simulink model "Rectifier_sim_model"  (R2016a)
settings: Solver=ode4  StartTime=0.0  StopTime=Tfinal  FixedStep=Ts  RelTol=1e-3
values from neighbouring files (symbols this model uses):
  Cdc = 15e-6    (= 1.5e-05)    [balancing_sim_parameters.m]    (also in rectifier_sim_parameters.m; sixthharmonicstudies_another_sim_param.m)
  Cdcrec = 4e-3    (= 0.004)    [balancing_sim_parameters.m]    (also in rectifier_sim_parameters.m = 0.0011; sixthharmonicstudies_another_sim_param.m)
  delta = 0    [balancing_sim_parameters.m]    (also in rectifier_sim_parameters.m; sixthharmonicstudies_another_sim_param.m = 2.09439510239)
  delta_third = 0*pi/180    (= 0)    [rectifier_sim_parameters.m]
  ESLrec = 100e-9    (= 1e-07)    [rectifier_sim_parameters.m]
  ESRrec = 10e-3    (= 0.01)    [rectifier_sim_parameters.m]
  f_third = 150    [rectifier_sim_parameters.m]
  GridFreq = 50    [balancing_sim_parameters.m]    (also in rectifier_sim_parameters.m; sixthharmonicstudies_another_sim_param.m)
  Is1_f = 150    [rectifier_sim_parameters.m]
  Is3_f = 150    [rectifier_sim_parameters.m]
  Isa1 = 10    [rectifier_sim_parameters.m]
  Isa1_delta = 0*pi/180    (= 0)    [rectifier_sim_parameters.m]
  Isa3 = third    (= 0)    [rectifier_sim_parameters.m]
  Isa3_delta = 0*pi/180    (= 0)    [rectifier_sim_parameters.m]
  Isb1 = 5    [rectifier_sim_parameters.m]
  Isb1_delta = -120*pi/180    (= -2.09439510239)    [rectifier_sim_parameters.m]
  Isb3 = third    (= 0)    [rectifier_sim_parameters.m]
  Isb3_delta = 0*pi/180    (= 0)    [rectifier_sim_parameters.m]
  Isc1 = 5    [rectifier_sim_parameters.m]
  Isc1_delta = 120*pi/180    (= 2.09439510239)    [rectifier_sim_parameters.m]
  Isc3 = third    (= 0)    [rectifier_sim_parameters.m]
  Isc3_delta = 0*pi/180    (= 0)    [rectifier_sim_parameters.m]
  Lload_1A = Lnom*1.00    [balancing_sim_parameters.m]    (also in rectifier_sim_parameters.m; sixthharmonicstudies_another_sim_param.m)
  Lload_1B = Lnom*1.00    [balancing_sim_parameters.m]    (also in rectifier_sim_parameters.m; sixthharmonicstudies_another_sim_param.m)
  Lload_1C = Lnom*1.00    [balancing_sim_parameters.m]    (also in rectifier_sim_parameters.m; sixthharmonicstudies_another_sim_param.m)
  Lmid = 1e-6    (= 1e-06)    [rectifier_sim_parameters.m]
  ma1 = 0.9    [balancing_sim_parameters.m]    (also in balancing_voltage_calc.m; rectifier_sim_parameters.m; sixthharmonicstudies_another_sim_param.m)
  ma_third = 0.5    [rectifier_sim_parameters.m]
  phase = [0 90 0 90]    [balancing_sim_parameters.m]    (also in rectifier_sim_parameters.m; sixthharmonicstudies_another_sim_param.m)
  Rin = 0    [balancing_sim_parameters.m]    (also in rectifier_sim_parameters.m = 10; sixthharmonicstudies_another_sim_param.m = 10)
  Ripth = 0.18    [balancing_sim_parameters.m]    (also in rectifier_sim_parameters.m; sixthharmonicstudies_another_sim_param.m)
  Rload_1A = Rnom*1.00    [balancing_sim_parameters.m]    (also in rectifier_sim_parameters.m; sixthharmonicstudies_another_sim_param.m)
  Rload_1B = Rnom*1.00    [balancing_sim_parameters.m]    (also in rectifier_sim_parameters.m; sixthharmonicstudies_another_sim_param.m = Rnom*2.5)
  Rload_1C = Rnom*1.00    [balancing_sim_parameters.m]    (also in rectifier_sim_parameters.m; sixthharmonicstudies_another_sim_param.m = Rnom*2.5)
  Rmid = 4    [balancing_sim_parameters.m]    (also in rectifier_sim_parameters.m = 3; sixthharmonicstudies_another_sim_param.m = 0.1)
  SA_delta1 = 0*pi/180    (= 0)    [rectifier_sim_parameters.m]
  SA_delta3 = 0*pi/180    (= 0)    [rectifier_sim_parameters.m]
  SA_f1 = 150    [rectifier_sim_parameters.m]
  SA_f3 = 150    [rectifier_sim_parameters.m]
  SA_ma1 = 0.9    [rectifier_sim_parameters.m]
  SA_ma3 = 0    [rectifier_sim_parameters.m]
  SB_delta3 = 0*pi/180    (= 0)    [rectifier_sim_parameters.m]
  SC_delta3 = 0*pi/180    (= 0)    [rectifier_sim_parameters.m]
  Ts = 1e-7    (= 1e-07)    [balancing_sim_parameters.m]    (also in rectifier_sim_parameters.m = 1e-06; sixthharmonicstudies_another_sim_param.m = 1e-06)
  Vacrms = 140    [balancing_sim_parameters.m]    (also in rectifier_sim_parameters.m = 120; sixthharmonicstudies_another_sim_param.m = 115)
  Vin = Vdc + Rin*(Pout/Vdc)+3    (= 1310.03703704)    [balancing_sim_parameters.m]    (also in rectifier_sim_parameters.m = 366.296296296; sixthharmonicstudies_another_sim_param.m = 344.814814815)
  wout = 2*pi*fout    (= 314.159265359)    [balancing_sim_parameters.m]    (also in rectifier_sim_parameters.m; sixthharmonicstudies_another_sim_param.m = 942.477796077)
undefined symbols (not defined in the file or in its folder): GridPhase, Lload, Rload, SA_delta, SA_f, SA_ma
libraries: powerlib x89, powerlib_meascontrol x63, simulink x6
settings Model: SimulationMode=accelerator  Creator=ugurm  LastModifiedBy=mesutto
settings DataIOCC: LimitDataPoints=on  SaveFormat=Array
settings DebuggingCC: UnderspecifiedInitializationDetection=Classic  MergeDetectMultiDrivingBlocksExec=none  SolverPrmCheckMsg=warning  StateNameClashWarn=warning
settings HardwareCC: ProdBitPerPointer=32  ProdLargestAtomicFloat=None  ProdIntDivRoundTo=Undefined  ProdEndianess=Unspecified  ProdWordSize=32  ProdHWDeviceType=32-bit Generic
settings ModelReferenceCC: PropagateSignalLabelsOutOfModel=off
settings ConfigComp: CovModelRefEnable=Off

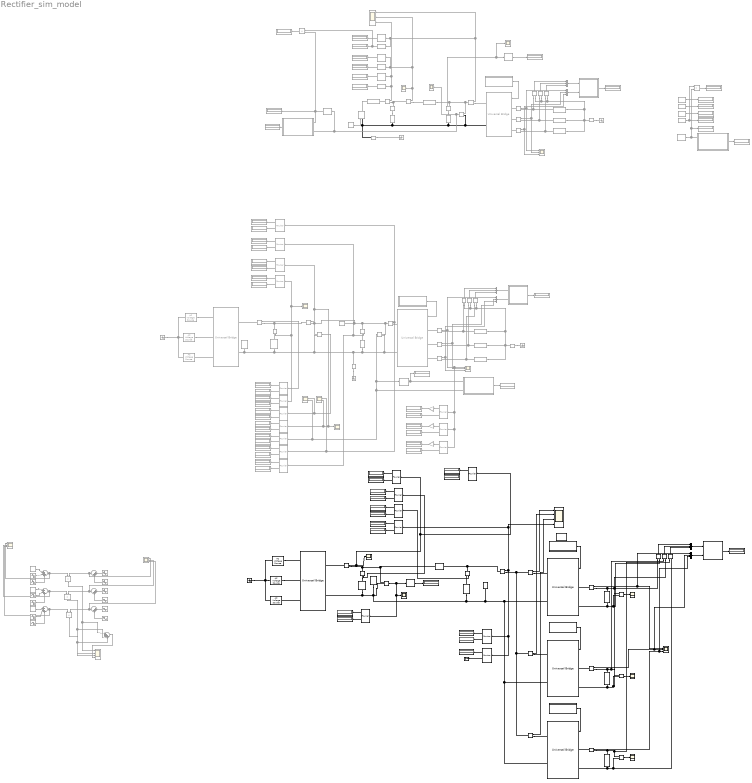
== system Rectifier_sim_model ==
  note: Iinput
  note: Idc
  note: Icap
  note: Vdc
  note: Vinput
  note: Ireccap
  note: Irec
  AC Voltage Source1 : powerlib/Electrical Sources/AC Voltage Source  Commented=on  Amplitude=Vacrms*sqrt(2)  Phase=-120  Frequency=GridFreq  SampleTime=0  Measurements=None  BusType=swing  Pref=10e3  Qref=0  Qmin=-inf  Qmax=+inf
  AC Voltage Source2 : powerlib/Electrical Sources/AC Voltage Source  Commented=on  Amplitude=Vacrms*sqrt(2)  Phase=0  Frequency=GridFreq  SampleTime=0  Measurements=None  BusType=swing  Pref=10e3  Qref=0  Qmin=-inf  Qmax=+inf
  AC Voltage Source3 : powerlib/Electrical Sources/AC Voltage Source  Commented=on  Amplitude=Vacrms*sqrt(2)  Phase=-240  Frequency=GridFreq  SampleTime=0  Measurements=None  BusType=swing  Pref=10e3  Qref=0  Qmin=-inf  Qmax=+inf
  AC Voltage Source4 : powerlib/Electrical Sources/AC Voltage Source  Amplitude=Vacrms*sqrt(2)  Phase=-120+GridPhase  Frequency=GridFreq  SampleTime=0  Measurements=None  BusType=swing  Pref=10e3  Qref=0  Qmin=-inf  Qmax=+inf
  AC Voltage Source5 : powerlib/Electrical Sources/AC Voltage Source  Amplitude=Vacrms*sqrt(2)  Phase=GridPhase  Frequency=GridFreq  SampleTime=0  Measurements=None  BusType=swing  Pref=10e3  Qref=0  Qmin=-inf  Qmax=+inf
  AC Voltage Source6 : powerlib/Electrical Sources/AC Voltage Source  Amplitude=Vacrms*sqrt(2)  Phase=-240+GridPhase  Frequency=GridFreq  SampleTime=0  Measurements=None  BusType=swing  Pref=10e3  Qref=0  Qmin=-inf  Qmax=+inf
  Constant : Constant  Commented=on  Value=1/2
  Constant1 : Constant  Commented=on  Value=Vin
  Constant2 : Constant  Commented=on  Value=1/2
  Constant3 : Constant  Commented=on  Value=1/2
  DC Voltage Source : powerlib/Electrical Sources/DC Voltage Source  Amplitude=270  Measurements=None
  Display{,1..48} (49 alike) : Display  Commented=on
  Display{49..65} (17 alike) : Display
  Fourier1 : powerlib_meascontrol/Measurements/Fourier  Commented=on  Freq=50  n=5  InInit=[0, 0]  Ts=0
  Fourier{8..11} (4 alike) : powerlib_meascontrol/Measurements/Fourier  Commented=on  Freq=9850  n=1  InInit=[0, 0]  Ts=0
  Fourier12 : powerlib_meascontrol/Measurements/Fourier  Commented=on  Freq=50  n=3  InInit=[0, 0]  Ts=0
  Fourier{2..6,13..14} (7 alike) : powerlib_meascontrol/Measurements/Fourier  Commented=on  Freq=50  n=6  InInit=[0, 0]  Ts=0
  Fourier{15,17..20,22} (6 alike) : powerlib_meascontrol/Measurements/Fourier  Freq=50  n=6  InInit=[0, 0]  Ts=0
  Fourier16 : powerlib_meascontrol/Measurements/Fourier  Freq=50  n=0  InInit=[0, 0]  Ts=0
  Fourier21 : powerlib_meascontrol/Measurements/Fourier  Freq=50  n=0  InInit=[0, 0]  Ts=0
  Fourier7 : powerlib_meascontrol/Measurements/Fourier  Commented=on  Freq=50  n=7  InInit=[0, 0]  Ts=0
  Gain : Gain  Commented=on  Gain=100
  Gain1 : Gain  Commented=on  Gain=100
  Gain2 : Gain  Commented=on  Gain=100
  Gate drive 1 : Subsystem  Commented=on
  Gate drive 2 : Subsystem
  Gate drive 3 : Subsystem
  Gate drive 4 : Subsystem
  Gate drive 5 : Subsystem  Commented=on
  Ground{1..3,5..6} (5 alike) : powerlib/Elements/Ground  Commented=on  LConnTagsString=a
  Ground4 : powerlib/Elements/Ground  LConnTagsString=a
  Idc_m{1..11,14..17,19} (16 alike) : powerlib/Measurements/Current Measurement  Commented=on  PhasorSimulation=off  OutputType=Complex  PSBequivalent=0
  Idc_m{12..13,18,20..26} (10 alike) : powerlib/Measurements/Current Measurement  PhasorSimulation=off  OutputType=Complex  PSBequivalent=0
  Mean{,1..7} (8 alike) : powerlib_meascontrol/Measurements/Mean  Commented=on  Freq=fout  Vinit=0  Ts=0
  Mean8 : powerlib_meascontrol/Measurements/Mean  Freq=50  Vinit=0  Ts=0
  Mux{,1..3} (4 alike) : Mux  Commented=on  Inputs=3
  Mux4 : Mux  Inputs=3
  Mux5 : Mux  Inputs=3
  Product{,1..4} (5 alike) : Product  Commented=on
  RMS{1..6} (6 alike) : powerlib_meascontrol/Measurements/RMS  Commented=on  TrueRMS=on  Freq=fout  RMSInit=0  Ts=0
  Scope{,2..5} (5 alike) : Scope  Commented=on
  Scope{1,6,8..10} (5 alike) : Scope  Commented=on  NumInputPorts=3
  Scope11 : Scope  Commented=on  NumInputPorts=2
  Scope12 : Scope  Commented=on  NumInputPorts=4
  Scope{13,16..19} (5 alike) : Scope
  Scope14 : Scope  NumInputPorts=3
  Scope15 : Scope  NumInputPorts=4
  Scope7 : Scope  Commented=on  NumInputPorts=2
  Series RLC Branch1 : powerlib/Elements/Series RLC Branch  Commented=on  LConnTagsString=__new0  RConnTagsString=__new0  BranchType=RL  Resistance=Rload_1B  Inductance=Lload_1B  SetiL0=off  InitialCurrent=0  Capacitance=1e-6  Setx0=off  InitialVoltage=0  Measurements=None
  Series RLC Branch{10,14,40,42} (4 alike) : powerlib/Elements/Series RLC Branch  Commented=on  LConnTagsString=__new0  RConnTagsString=__new0  BranchType=R  Resistance=1e12  Inductance=Lload  SetiL0=off  InitialCurrent=0  Capacitance=1e-6  Setx0=off  InitialVoltage=0  Measurements=None
  Series RLC Branch11 : powerlib/Elements/Series RLC Branch  Commented=on  LConnTagsString=__new0  RConnTagsString=__new0  BranchType=RL  Resistance=Rload_1A  Inductance=Lload_1A  SetiL0=off  InitialCurrent=0  Capacitance=1e-6  Setx0=off  InitialVoltage=0  Measurements=None
  Series RLC Branch12 : powerlib/Elements/Series RLC Branch  Commented=on  LConnTagsString=__new0  RConnTagsString=__new0  BranchType=C  Resistance=Rload  Inductance=Lload  SetiL0=off  InitialCurrent=0  Capacitance=Cdc  Setx0=off  InitialVoltage=0  Measurements=None
  Series RLC Branch13 : powerlib/Elements/Series RLC Branch  Commented=on  LConnTagsString=__new0  RConnTagsString=__new0  BranchType=RL  Resistance=Rmid  Inductance=Lmid  SetiL0=off  InitialCurrent=0  Capacitance=1e-6  Setx0=off  InitialVoltage=0  Measurements=None
  Series RLC Branch15 : powerlib/Elements/Series RLC Branch  LConnTagsString=__new0  RConnTagsString=__new0  BranchType=RL  Resistance=Rload_1A  Inductance=Lload_1A  SetiL0=off  InitialCurrent=0  Capacitance=1e-6  Setx0=off  InitialVoltage=0  Measurements=None
  Series RLC Branch16 : powerlib/Elements/Series RLC Branch  LConnTagsString=__new0  RConnTagsString=__new0  BranchType=R  Resistance=Rmid  Inductance=1e-6  SetiL0=off  InitialCurrent=0  Capacitance=Cdcrec  Setx0=on  InitialVoltage=270  Measurements=None
  Series RLC Branch17 : powerlib/Elements/Series RLC Branch  LConnTagsString=__new0  RConnTagsString=__new0  BranchType=C  Resistance=ESRrec  Inductance=ESLrec  SetiL0=off  InitialCurrent=0  Capacitance=Cdc  Setx0=off  InitialVoltage=270  Measurements=None
  Series RLC Branch18 : powerlib/Elements/Series RLC Branch  LConnTagsString=__new0  RConnTagsString=__new0  BranchType=R  Resistance=36.5  Inductance=ESLrec  SetiL0=off  InitialCurrent=0  Capacitance=Cdcrec  Setx0=on  InitialVoltage=270  Measurements=None
  Series RLC Branch19 : powerlib/Elements/Series RLC Branch  LConnTagsString=__new0  RConnTagsString=__new0  BranchType=C  Resistance=ESRrec  Inductance=ESLrec  SetiL0=off  InitialCurrent=0  Capacitance=Cdcrec  Setx0=on  InitialVoltage=270  Measurements=None
  Series RLC Branch2 : powerlib/Elements/Series RLC Branch  Commented=on  LConnTagsString=__new0  RConnTagsString=__new0  BranchType=RL  Resistance=Rload_1C  Inductance=Lload_1C  SetiL0=off  InitialCurrent=0  Capacitance=1e-6  Setx0=off  InitialVoltage=0  Measurements=None
  Series RLC Branch20 : powerlib/Elements/Series RLC Branch  Commented=on  LConnTagsString=__new0  RConnTagsString=__new0  BranchType=R  Resistance=Rin  Inductance=1e-3  SetiL0=off  InitialCurrent=0  Capacitance=1e-6  Setx0=off  InitialVoltage=0  Measurements=None
  Series RLC Branch21 : powerlib/Elements/Series RLC Branch  Commented=on  LConnTagsString=__new0  RConnTagsString=__new0  BranchType=C  Resistance=Rload  Inductance=Lload  SetiL0=off  InitialCurrent=0  Capacitance=Cdc  Setx0=off  InitialVoltage=0  Measurements=None
  Series RLC Branch22 : powerlib/Elements/Series RLC Branch  LConnTagsString=__new0  RConnTagsString=__new0  BranchType=RL  Resistance=Rload_1A  Inductance=Lload_1A  SetiL0=off  InitialCurrent=0  Capacitance=1e-6  Setx0=off  InitialVoltage=0  Measurements=None
  Series RLC Branch23 : powerlib/Elements/Series RLC Branch  LConnTagsString=__new0  RConnTagsString=__new0  BranchType=RL  Resistance=Rload_1A  Inductance=Lload_1A  SetiL0=off  InitialCurrent=0  Capacitance=1e-6  Setx0=off  InitialVoltage=0  Measurements=None
  Series RLC Branch3 : powerlib/Elements/Series RLC Branch  Commented=on  LConnTagsString=__new0  RConnTagsString=__new0  BranchType=C  Resistance=Rload  Inductance=Lload  SetiL0=off  InitialCurrent=0  Capacitance=Cdcrec  Setx0=on  InitialVoltage=270  Measurements=None
  Series RLC Branch4 : powerlib/Elements/Series RLC Branch  Commented=on  LConnTagsString=__new0  RConnTagsString=__new0  BranchType=R  Resistance=Rmid  Inductance=1e-3  SetiL0=off  InitialCurrent=0  Capacitance=1e-6  Setx0=off  InitialVoltage=0  Measurements=None
  Series RLC Branch5 : powerlib/Elements/Series RLC Branch  Commented=on  LConnTagsString=__new0  RConnTagsString=__new0  BranchType=RLC  Resistance=ESRrec  Inductance=ESLrec  SetiL0=off  InitialCurrent=0  Capacitance=Cdcrec  Setx0=on  InitialVoltage=270  Measurements=None
  Series RLC Branch6 : powerlib/Elements/Series RLC Branch  Commented=on  LConnTagsString=__new0  RConnTagsString=__new0  BranchType=RL  Resistance=Rload_1A  Inductance=Lload_1A  SetiL0=off  InitialCurrent=0  Capacitance=1e-6  Setx0=off  InitialVoltage=0  Measurements=None
  Series RLC Branch7 : powerlib/Elements/Series RLC Branch  Commented=on  LConnTagsString=__new0  RConnTagsString=__new0  BranchType=C  Resistance=ESRrec  Inductance=ESLrec  SetiL0=off  InitialCurrent=0  Capacitance=Cdcrec  Setx0=on  InitialVoltage=270  Measurements=None
  Series RLC Branch8 : powerlib/Elements/Series RLC Branch  Commented=on  LConnTagsString=__new0  RConnTagsString=__new0  BranchType=RL  Resistance=Rload_1B  Inductance=Lload_1B  SetiL0=off  InitialCurrent=0  Capacitance=1e-6  Setx0=off  InitialVoltage=0  Measurements=None
  Series RLC Branch9 : powerlib/Elements/Series RLC Branch  Commented=on  LConnTagsString=__new0  RConnTagsString=__new0  BranchType=RL  Resistance=Rload_1C  Inductance=Lload_1C  SetiL0=off  InitialCurrent=0  Capacitance=1e-6  Setx0=off  InitialVoltage=0  Measurements=None
  Sine Wave : Sin  Commented=on  Amplitude=Isa1  Frequency=Is1_f*2*pi  Phase=Isa1_delta  SampleTime=0
  Sine Wave1 : Sin  Commented=on  Amplitude=SA_ma1/2  Frequency=SA_f1*2*pi  Phase=SA_delta1  SampleTime=0
  Sine Wave10 : Sin  Commented=on  Amplitude=SA_ma3/2  Frequency=SA_f3*2*pi  Phase=SB_delta3  SampleTime=0
  Sine Wave11 : Sin  Commented=on  Amplitude=SA_ma3/2  Frequency=SA_f3*2*pi  Phase=SC_delta3  SampleTime=0
  Sine Wave2 : Sin  Commented=on  Amplitude=SA_ma1/2  Frequency=SA_f1*2*pi  Phase=SA_delta1-2*pi/3  SampleTime=0
  Sine Wave3 : Sin  Commented=on  Amplitude=Isa3  Frequency=Is3_f*2*pi  Phase=Isa3_delta  SampleTime=0
  Sine Wave4 : Sin  Commented=on  Amplitude=SA_ma/2  Frequency=SA_f*2*pi  Phase=SA_delta+2*pi/3  SampleTime=0
  Sine Wave5 : Sin  Commented=on  Amplitude=Isb1  Frequency=Is1_f*2*pi  Phase=Isb1_delta  SampleTime=0
  Sine Wave6 : Sin  Commented=on  Amplitude=Isb3  Frequency=Is3_f*2*pi  Phase=Isb3_delta  SampleTime=0
  Sine Wave7 : Sin  Commented=on  Amplitude=Isc1  Frequency=Is1_f*2*pi  Phase=Isc1_delta  SampleTime=0
  Sine Wave8 : Sin  Commented=on  Amplitude=Isc3  Frequency=Is3_f*2*pi  Phase=Isc3_delta  SampleTime=0
  Sine Wave9 : Sin  Commented=on  Amplitude=SA_ma3/2  Frequency=SA_f3*2*pi  Phase=SA_delta3  SampleTime=0
  Subsystem1 : Subsystem  Commented=on
  Subsystem2 : Subsystem  Commented=on
  Subsystem3 : Subsystem  Commented=on
  Subsystem4 : Subsystem  Commented=on
  Subsystem5 : Subsystem  Commented=on
  Subsystem6 : Subsystem
  Sum{1..2,4,7} (4 alike) : Sum  Commented=on  Inputs=|+++
  Sum3 : Sum  Commented=on  Inputs=|++
  Sum5 : Sum  Commented=on  Inputs=|++
  Sum6 : Sum  Commented=on  Inputs=|++
  Terminator : Terminator
  Universal Bridge1 : powerlib/Power Electronics/Universal Bridge  Commented=on  Arms=3  SnubberResistance=1e5  SnubberCapacitance=inf  Device=Diodes  Ron=1e-6  Lon=0  ForwardVoltages="[  0  0  ]"  ForwardVoltage=0  GTOparameters=[ 10e-6 , 20e-6 ]  IGBTparameters=[0,0]  Measurements=None  Measurements_2=None  converterType=Rectifier
  Universal Bridge2 : powerlib/Power Electronics/Universal Bridge  Commented=on  Arms=3  SnubberResistance=1e5  SnubberCapacitance=inf  Device=IGBT / Diodes  Ron=1e-6  Lon=0  ForwardVoltages="[  0  0  ]"  ForwardVoltage=0  GTOparameters=[ 10e-6 , 20e-6 ]  IGBTparameters=[0,0]  Measurements=None  Measurements_2=None  converterType=Rectifier
  Universal Bridge3 : powerlib/Power Electronics/Universal Bridge  Arms=2  SnubberResistance=1e5  SnubberCapacitance=inf  Device=IGBT / Diodes  Ron=1e-6  Lon=0  ForwardVoltages="[  0  0  ]"  ForwardVoltage=0  GTOparameters=[ 10e-6 , 20e-6 ]  IGBTparameters=[0,0]  Measurements=None  Measurements_2=None  converterType=Rectifier
  Universal Bridge4 : powerlib/Power Electronics/Universal Bridge  Commented=on  Arms=3  SnubberResistance=1e5  SnubberCapacitance=inf  Device=IGBT / Diodes  Ron=1e-6  Lon=0  ForwardVoltages="[  0  0  ]"  ForwardVoltage=0  GTOparameters=[ 10e-6 , 20e-6 ]  IGBTparameters=[0,0]  Measurements=None  Measurements_2=None  converterType=Rectifier
  Universal Bridge5 : powerlib/Power Electronics/Universal Bridge  Arms=2  SnubberResistance=1e5  SnubberCapacitance=inf  Device=IGBT / Diodes  Ron=1e-6  Lon=0  ForwardVoltages="[  0  0  ]"  ForwardVoltage=0  GTOparameters=[ 10e-6 , 20e-6 ]  IGBTparameters=[0,0]  Measurements=None  Measurements_2=None  converterType=Rectifier
  Universal Bridge6 : powerlib/Power Electronics/Universal Bridge  Arms=2  SnubberResistance=1e5  SnubberCapacitance=inf  Device=IGBT / Diodes  Ron=1e-6  Lon=0  ForwardVoltages="[  0  0  ]"  ForwardVoltage=0  GTOparameters=[ 10e-6 , 20e-6 ]  IGBTparameters=[0,0]  Measurements=None  Measurements_2=None  converterType=Rectifier
  Universal Bridge7 : powerlib/Power Electronics/Universal Bridge  Arms=3  SnubberResistance=1e5  SnubberCapacitance=inf  Device=Diodes  Ron=1e-6  Lon=0  ForwardVoltages="[  0  0  ]"  ForwardVoltage=0  GTOparameters=[ 10e-6 , 20e-6 ]  IGBTparameters=[0,0]  Measurements=None  Measurements_2=None  converterType=Rectifier
  Vdc1 : powerlib/Electrical Sources/Controlled Voltage Source  Commented=on  Initialize=off  Source_Type=DC  Amplitude=200  Phase=0  Frequency=0  Measurements=None
  Vdc_m{1..9} (9 alike) : powerlib/Measurements/Voltage Measurement  Commented=on  PhasorSimulation=off  OutputType=Complex  PSBequivalent=0
  Vdc_m{10..15} (6 alike) : powerlib/Measurements/Voltage Measurement  PhasorSimulation=off  OutputType=Complex  PSBequivalent=0
  Voltage Measurement : powerlib/Measurements/Voltage Measurement  PhasorSimulation=off  OutputType=Complex  PSBequivalent=0
  powergui1 : powerlib/powergui  Priority=1  SimulationMode=Discrete  SolverType=Tustin  SampleTime=Ts  frequency=60  SPID=off  DisableSnubberDevices=off  DisableRonSwitches=off  DisableVfSwitches=off  SwTol=0  DisplayEquations=off  Interpol=off  ExternalGateDelay=off  methode=off  Ts=0  FunctionMessages=off  echomessages=off  HookPort=off  EnableUseOfTLC=off  x0status=blocks  frequencyindice=0  Pbase=100e6  ErrMax=1e-4  Iterations=50  UnitsV=kV  UnitsW=MW  buscounter=0  RestoreLinks=warning  ResistiveCurrentMeasurement=off  Frange=[0:2:500]  Ylog=off  Xlog=on  ShowGrid=off  save=off  variable=ZData  structure=newidcs  ZoomFFT=off  StartTime=0.04  cycles=5  DisplayStyle=5  fundamental=50  FreqAxis=off  MaxFrequency=2000  frequencyindicesteady=1  RmsSteady=1  display=off
  wires:
  Gate drive 5/1(gate1) -> Universal Bridge4/1
  Idc_m14/1 -> Mux1/1, Scope8/1
  Constant1/1 -> Vdc1/1
  Idc_m15/1 -> RMS3/1, Scope3/1
  Idc_m16/1 -> Mux1/2, Scope8/2
  Idc_m17/1 -> Scope8/3, Mux1/3
  RMS3/1 -> Display/1
  Mean/1 -> Product/2, Subsystem5/1(Vdcavg), Display8/1
  RMS2/1 -> Display4/1
  Idc_m11/1 -> Scope1/1, RMS2/1, Mean3/1
  Idc_m19/1 -> Scope2/1, Scope1/2, Mean6/1, RMS5/1
  Mean3/1 -> Product/1, Display7/1
  RMS5/1 -> Display12/1
  Mean6/1 -> Display11/1
  Subsystem5/1(Out1) -> Display14/1
  Product/1 -> Display17/1
  Vdc_m5/1 -> Mux/1
  Vdc_m2/1 -> Mux/2
  Vdc_m6/1 -> Mux/3
  Mux/1 -> Subsystem4/1(Vabc)
  Mux1/1 -> Subsystem4/2(Iabc)
  Subsystem4/1(Poutp) -> Display20/1
  Vdc_m1/1 -> Scope4/1, Mean/1, Subsystem5/2(vdc)
  Idc_m2/1 -> Mean1/1, Scope1/3, RMS1/1
  Mean1/1 -> Display1/1
  RMS1/1 -> Display2/1
  Idc_m4/1 -> Fourier9/1, Scope11/2, Fourier3/1, Scope/1
  Vdc_m3/1 -> Fourier2/1, Scope7/1
  Mean5/1 -> Display15/1, Product1/2, Subsystem1/1(Vdcavg)
  Subsystem1/1(Out1) -> Display3/1
  RMS4/1 -> Display5/1
  Mean2/1 -> Display6/1
  Mean4/1 -> Product1/1, Display10/1
  RMS6/1 -> Display9/1
  Product1/1 -> Display13/1
  Gate drive 1/1(gate1) -> Universal Bridge2/1
  Idc_m6/1 -> Mux3/1, Fourier12/1, Fourier7/1, Fourier1/1, Scope9/1
  Idc_m7/1 -> Mux3/2, Scope9/2
  Idc_m8/1 -> Mux3/3, Scope9/3
  Vdc_m8/1 -> Mux2/1
  Vdc_m7/1 -> Mux2/2
  Vdc_m9/1 -> Mux2/3
  Mux2/1 -> Subsystem2/1(Vabc)
  Mux3/1 -> Subsystem2/2(Iabc)
  Subsystem2/1(Poutp) -> Display18/1
  Vdc_m4/1 -> Fourier4/1, Scope7/2, Subsystem3/2(vdc), Mean7/1
  Mean7/1 -> Subsystem3/1(Vdcavg), Display16/1
  Subsystem3/1(Out1) -> Display19/1
  Fourier2/1 -> Display25/1
  Fourier2/2 -> Display26/1
  Fourier3/1 -> Display27/1
  Fourier3/2 -> Display28/1
  Fourier4/1 -> Display29/1
  Fourier4/2 -> Display30/1
  Fourier5/1 -> Display31/1
  Fourier5/2 -> Display32/1
  Fourier6/1 -> Display33/1
  Fourier6/2 -> Display34/1
  Fourier1/1 -> Gain/1
  Fourier1/2 -> Display22/1
  Fourier7/1 -> Gain1/1
  Fourier7/2 -> Display24/1
  Fourier8/1 -> Display35/1
  Fourier8/2 -> Display36/1
  Fourier9/1 -> Display37/1
  Fourier9/2 -> Display38/1
  Idc_m10/1 -> Fourier10/1, Fourier6/1
  Fourier10/1 -> Display39/1
  Fourier10/2 -> Display40/1
  Idc_m5/1 -> Fourier5/1, Scope11/1, Fourier11/1
  Fourier11/1 -> Display41/1
  Fourier11/2 -> Display42/1
  Fourier12/1 -> Gain2/1
  Fourier12/2 -> Display44/1
  Gain/1 -> Display21/1
  Gain1/1 -> Display23/1
  Gain2/1 -> Display43/1
  Idc_m3/1 -> Scope5/1, Fourier8/1, Fourier14/1
  Idc_m9/1 -> Fourier13/1
  Fourier13/1 -> Display45/1
  Fourier13/2 -> Display46/1
  Fourier14/1 -> Display47/1
  Fourier14/2 -> Display48/1
  Sine Wave/1 -> Sum3/1
  Sine Wave3/1 -> Sum3/2
  Constant/1 -> Sum1/1
  Sine Wave1/1 -> Sum1/2
  Constant2/1 -> Sum2/1
  Sine Wave2/1 -> Sum2/2
  Constant3/1 -> Sum4/1
  Sine Wave4/1 -> Sum4/2
  Sine Wave5/1 -> Sum5/1
  Sine Wave6/1 -> Sum5/2
  Sine Wave7/1 -> Sum6/1
  Sine Wave8/1 -> Sum6/2
  Sum2/1 -> Product3/1, Scope6/2
  Sum1/1 -> Product2/1, Scope6/1
  Sum5/1 -> Product3/2, Scope10/2
  Sum3/1 -> Product2/2, Scope10/1
  Sum4/1 -> Product4/1, Scope6/3
  Sum6/1 -> Product4/2, Scope10/3
  Product2/1 -> Sum7/1, Scope12/1
  Product3/1 -> Scope12/2, Sum7/2
  Product4/1 -> Scope12/3, Sum7/3
  Sum7/1 -> Scope12/4
  Sine Wave9/1 -> Sum1/3
  Sine Wave10/1 -> Sum2/3
  Sine Wave11/1 -> Sum4/3
  Gate drive 2/1(gate1) -> Universal Bridge3/1
  Vdc_m10/1 -> Scope13/1
  Gate drive 3/1(gate1) -> Universal Bridge5/1
  Vdc_m11/1 -> Scope16/1
  Gate drive 4/1(gate1) -> Universal Bridge6/1
  Vdc_m12/1 -> Scope18/1
  Idc_m13/1 -> Scope15/1
  Idc_m21/1 -> Scope15/2
  Idc_m22/1 -> Scope15/3
  Idc_m23/1 -> Scope15/4, Fourier19/1, Fourier16/1, Fourier15/1
  Fourier15/1 -> Display49/1
  Fourier15/2 -> Display50/1
  Fourier16/1 -> Display51/1
  Fourier16/2 -> Terminator/1
  Fourier17/1 -> Display52/1
  Fourier17/2 -> Display53/1
  Fourier18/1 -> Display54/1
  Fourier18/2 -> Display55/1
  Voltage Measurement/1 -> Mean8/1, Scope19/1, Fourier18/1
  Mean8/1 -> Display56/1
  Fourier19/1 -> Display57/1
  Fourier19/2 -> Display58/1
  Idc_m25/1 -> Fourier20/1
  Fourier20/1 -> Display59/1
  Fourier20/2 -> Display60/1
  Fourier21/1 -> Display61/1
  Idc_m24/1 -> Scope17/1, Fourier21/1, Fourier17/1
  Idc_m12/1 -> Mux5/1, Scope14/1
  Idc_m18/1 -> Mux5/2, Scope14/2
  Idc_m20/1 -> Scope14/3, Mux5/3
  Vdc_m14/1 -> Mux4/1
  Vdc_m13/1 -> Mux4/2
  Vdc_m15/1 -> Mux4/3
  Mux4/1 -> Subsystem6/1(Vabc)
  Mux5/1 -> Subsystem6/2(Iabc)
  Subsystem6/1(Poutp) -> Display63/1
  Idc_m26/1 -> Fourier22/1
  Fourier22/2 -> Display65/1
  Fourier22/1 -> Display64/1
  connections:
  Vdc_m5/LConn1 -- Series RLC Branch6/LConn1 -- Idc_m14/RConn1
  Series RLC Branch42/RConn1 -- Ground6/LConn1
  Series RLC Branch40/RConn1 -- Ground5/LConn1
  Idc_m14/LConn1 -- Universal Bridge4/LConn1
  Idc_m15/LConn1 -- Series RLC Branch21/LConn1
  Vdc1/RConn1 -- Series RLC Branch20/LConn1
  Series RLC Branch42/LConn1 -- Vdc_m5/LConn2 -- Vdc_m2/LConn2 -- Vdc_m6/LConn2 -- Series RLC Branch6/RConn1 -- Series RLC Branch1/RConn1 -- Series RLC Branch2/RConn1
  Idc_m16/LConn1 -- Universal Bridge4/LConn2
  Idc_m17/LConn1 -- Universal Bridge4/LConn3
  Series RLC Branch2/LConn1 -- Vdc_m6/LConn1 -- Idc_m17/RConn1
  Series RLC Branch1/LConn1 -- Vdc_m2/LConn1 -- Idc_m16/RConn1
  Idc_m15/RConn1 -- Series RLC Branch4/RConn1 -- Vdc_m1/LConn1 -- Idc_m11/LConn1
  Idc_m11/RConn1 -- Universal Bridge4/RConn1
  Idc_m19/LConn1 -- Idc_m2/RConn1 -- Idc_m1/RConn1
  Vdc_m1/LConn2 -- Universal Bridge4/RConn2 -- Series RLC Branch21/RConn1 -- Series RLC Branch3/RConn1 -- Vdc1/LConn1 -- Series RLC Branch40/LConn1
  Idc_m1/LConn1 -- Series RLC Branch3/LConn1
  Idc_m2/LConn1 -- Series RLC Branch20/RConn1
  Idc_m19/RConn1 -- Series RLC Branch4/LConn1
  Universal Bridge1/LConn3 -- AC Voltage Source3/RConn1
  AC Voltage Source2/RConn1 -- Universal Bridge1/LConn1
  Ground1/LConn1 -- AC Voltage Source2/LConn1 -- AC Voltage Source3/LConn1 -- AC Voltage Source1/LConn1
  Idc_m4/LConn1 -- Idc_m9/RConn1 -- Idc_m3/LConn1
  Universal Bridge2/RConn2 -- Vdc_m4/LConn2 -- Series RLC Branch12/RConn1 -- Series RLC Branch14/LConn1 -- Series RLC Branch7/RConn1 -- Series RLC Branch5/RConn1 -- Universal Bridge1/RConn2 -- Vdc_m3/LConn2
  Vdc_m8/LConn1 -- Series RLC Branch11/LConn1 -- Idc_m6/RConn1
  Series RLC Branch9/RConn1 -- Vdc_m8/LConn2 -- Vdc_m7/LConn2 -- Vdc_m9/LConn2 -- Series RLC Branch11/RConn1 -- Series RLC Branch8/RConn1 -- Series RLC Branch10/LConn1
  Series RLC Branch9/LConn1 -- Vdc_m9/LConn1 -- Idc_m8/RConn1
  Series RLC Branch8/LConn1 -- Vdc_m7/LConn1 -- Idc_m7/RConn1
  Idc_m6/LConn1 -- Universal Bridge2/LConn1
  Idc_m5/RConn1 -- Universal Bridge2/RConn1
  Series RLC Branch10/RConn1 -- Ground2/LConn1
  Idc_m8/LConn1 -- Universal Bridge2/LConn3
  Idc_m7/LConn1 -- Universal Bridge2/LConn2
  Idc_m10/RConn1 -- Series RLC Branch12/LConn1
  Vdc_m3/LConn1 -- Idc_m4/RConn1 -- Vdc_m4/LConn1 -- Idc_m5/LConn1 -- Idc_m10/LConn1 -- Series RLC Branch13/RConn1
  Series RLC Branch14/RConn1 -- Ground3/LConn1
  AC Voltage Source1/RConn1 -- Universal Bridge1/LConn2
  Series RLC Branch7/LConn1 -- Idc_m3/RConn1
  Idc_m9/LConn1 -- Universal Bridge1/RConn1
  Idc_m12/RConn1 -- Series RLC Branch22/LConn1 -- Vdc_m14/LConn1 -- Vdc_m10/LConn2
  Idc_m12/LConn1 -- Universal Bridge3/LConn1
  Idc_m13/RConn1 -- Universal Bridge3/RConn1
  Idc_m13/LConn1 -- Idc_m23/RConn1 -- Idc_m22/LConn1 -- Idc_m21/LConn1
  Idc_m18/RConn1 -- Series RLC Branch15/LConn1 -- Vdc_m13/LConn1 -- Vdc_m11/LConn2
  Idc_m18/LConn1 -- Universal Bridge5/LConn1
  Idc_m20/RConn1 -- Series RLC Branch23/LConn1 -- Vdc_m15/LConn1 -- Vdc_m12/LConn2
  Vdc_m12/LConn1 -- Vdc_m15/LConn2 -- Series RLC Branch23/RConn1 -- Universal Bridge6/LConn2
  Idc_m20/LConn1 -- Universal Bridge6/LConn1
  Idc_m21/RConn1 -- Universal Bridge5/RConn1
  Idc_m22/RConn1 -- Universal Bridge6/RConn1
  Vdc_m10/LConn1 -- Series RLC Branch22/RConn1 -- Universal Bridge3/LConn2 -- Vdc_m14/LConn2
  Vdc_m11/LConn1 -- Vdc_m13/LConn2 -- Series RLC Branch15/RConn1 -- Universal Bridge5/LConn2
  AC Voltage Source4/LConn1 -- Ground4/LConn1 -- AC Voltage Source5/LConn1 -- AC Voltage Source6/LConn1
  Universal Bridge3/RConn2 -- Universal Bridge6/RConn2 -- Universal Bridge5/RConn2 -- Series RLC Branch17/RConn1 -- Series RLC Branch18/RConn1 -- Voltage Measurement/LConn2 -- Universal Bridge7/RConn2 -- Series RLC Branch19/RConn1 -- DC Voltage Source/LConn1
  AC Voltage Source5/RConn1 -- Universal Bridge7/LConn1
  Universal Bridge7/LConn3 -- AC Voltage Source6/RConn1
  AC Voltage Source4/RConn1 -- Universal Bridge7/LConn2
  Idc_m24/LConn1 -- Universal Bridge7/RConn1
  Idc_m24/RConn1 -- Idc_m25/LConn1 -- Series RLC Branch16/RConn1 -- Voltage Measurement/LConn1
  Idc_m23/LConn1 -- Idc_m26/LConn1 -- Series RLC Branch16/LConn1
  Idc_m25/RConn1 -- Series RLC Branch19/LConn1
  Idc_m26/RConn1 -- Series RLC Branch17/LConn1

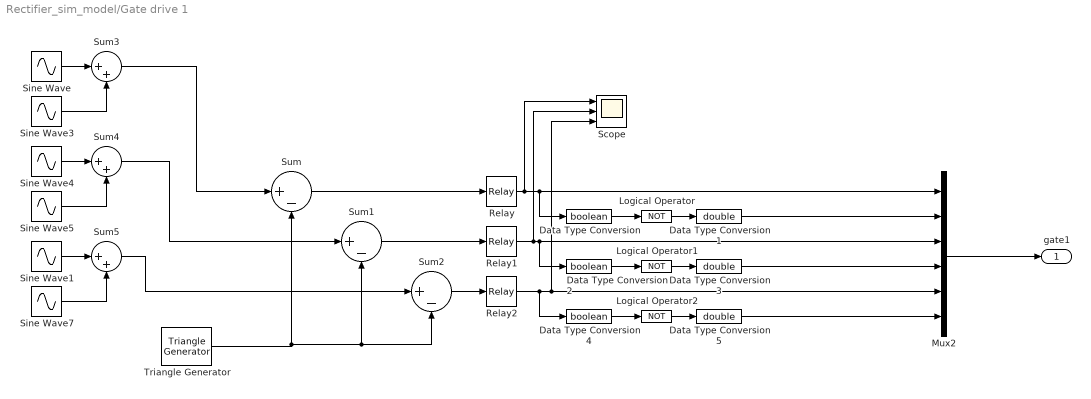
== system Rectifier_sim_model/Gate drive 1 ==
  Data Type Conversion : DataTypeConversion  OutDataTypeStr=boolean
  Data Type Conversion1 : DataTypeConversion  OutDataTypeStr=double
  Data Type Conversion2 : DataTypeConversion  OutDataTypeStr=boolean
  Data Type Conversion3 : DataTypeConversion  OutDataTypeStr=double
  Data Type Conversion4 : DataTypeConversion  OutDataTypeStr=boolean
  Data Type Conversion5 : DataTypeConversion  OutDataTypeStr=double
  Logical Operator : Logic  Operator=NOT  AllPortsSameDT=off  OutDataTypeStr=boolean
  Logical Operator1 : Logic  Operator=NOT  AllPortsSameDT=off  OutDataTypeStr=boolean
  Logical Operator2 : Logic  Operator=NOT  AllPortsSameDT=off  OutDataTypeStr=boolean
  Mux2 : Mux  Inputs=6
  Relay : Relay
  Relay1 : Relay
  Relay2 : Relay
  Scope : Scope  NumInputPorts=3
  Sine Wave : Sin  Amplitude=ma1  Frequency=wout  Phase=delta  SampleTime=0
  Sine Wave1 : Sin  Amplitude=ma1  Frequency=wout  Phase=2*pi/3+delta  SampleTime=0
  Sine Wave3 : Sin  Amplitude=ma_third  Frequency=f_third*2*pi  Phase=delta_third  SampleTime=0
  Sine Wave4 : Sin  Amplitude=ma1  Frequency=wout  Phase=-2*pi/3+delta  SampleTime=0
  Sine Wave5 : Sin  Amplitude=ma_third  Frequency=f_third*2*pi  Phase=delta_third  SampleTime=0
  Sine Wave7 : Sin  Amplitude=ma_third  Frequency=f_third*2*pi  Phase=delta_third  SampleTime=0
  Sum : Sum  Inputs=|+-
  Sum1 : Sum  Inputs=|+-
  Sum2 : Sum  Inputs=|+-
  Sum3 : Sum  Inputs=|++
  Sum4 : Sum  Inputs=|++
  Sum5 : Sum  Inputs=|++
  Triangle Generator : powerlib_meascontrol/Pulse & Signal Generators/Triangle Generator  Freq=fsw  Phase=phase(1)  Ts=Ts
  gate1 : Outport
  wires:
  Triangle Generator/1 -> Sum1/2, Sum2/2, Sum/2
  Sum4/1 -> Sum1/1
  Sum5/1 -> Sum2/1
  Sum/1 -> Relay/1
  Sum1/1 -> Relay1/1
  Sum2/1 -> Relay2/1
  Data Type Conversion/1 -> Logical Operator/1
  Relay/1 -> Scope/1, Data Type Conversion/1, Mux2/1
  Logical Operator/1 -> Data Type Conversion1/1
  Data Type Conversion1/1 -> Mux2/2
  Data Type Conversion2/1 -> Logical Operator1/1
  Relay1/1 -> Scope/2, Data Type Conversion2/1, Mux2/3
  Logical Operator1/1 -> Data Type Conversion3/1
  Data Type Conversion3/1 -> Mux2/4
  Data Type Conversion4/1 -> Logical Operator2/1
  Relay2/1 -> Scope/3, Mux2/5, Data Type Conversion4/1
  Logical Operator2/1 -> Data Type Conversion5/1
  Data Type Conversion5/1 -> Mux2/6
  Mux2/1 -> gate1/1
  Sine Wave/1 -> Sum3/1
  Sine Wave3/1 -> Sum3/2
  Sum3/1 -> Sum/1
  Sine Wave4/1 -> Sum4/1
  Sine Wave5/1 -> Sum4/2
  Sine Wave1/1 -> Sum5/1
  Sine Wave7/1 -> Sum5/2

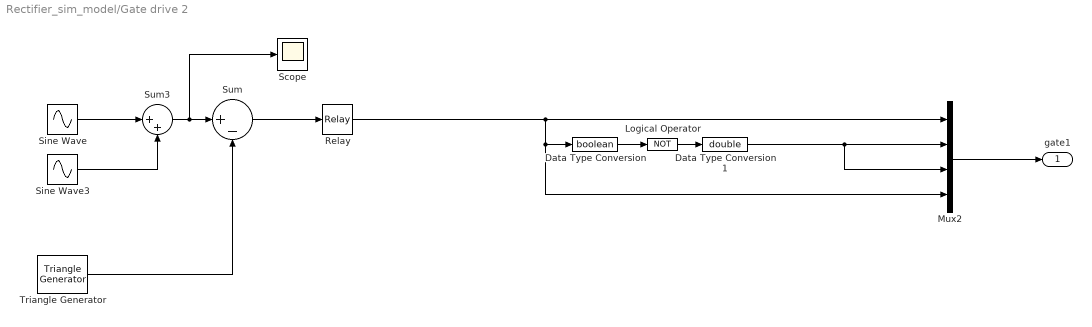
== system Rectifier_sim_model/Gate drive 2 ==
  Data Type Conversion : DataTypeConversion  OutDataTypeStr=boolean
  Data Type Conversion1 : DataTypeConversion  OutDataTypeStr=double
  Logical Operator : Logic  Operator=NOT  AllPortsSameDT=off  OutDataTypeStr=boolean
  Mux2 : Mux
  Relay : Relay
  Scope : Scope
  Sine Wave : Sin  Amplitude=ma1  Frequency=wout  Phase=delta  SampleTime=0
  Sine Wave3 : Sin  Amplitude=ma_third  Frequency=f_third*2*pi  Phase=delta_third  SampleTime=0
  Sum : Sum  Inputs=|+-
  Sum3 : Sum  Inputs=|++
  Triangle Generator : powerlib_meascontrol/Pulse & Signal Generators/Triangle Generator  Freq=10000  Phase=0  Ts=Ts
  gate1 : Outport
  wires:
  Sum3/1 -> Scope/1, Sum/1
  Sine Wave3/1 -> Sum3/2
  Sine Wave/1 -> Sum3/1
  Mux2/1 -> gate1/1
  Data Type Conversion1/1 -> Mux2/3, Mux2/2
  Logical Operator/1 -> Data Type Conversion1/1
  Data Type Conversion/1 -> Logical Operator/1
  Sum/1 -> Relay/1
  Triangle Generator/1 -> Sum/2
  Relay/1 -> Mux2/1, Data Type Conversion/1, Mux2/4

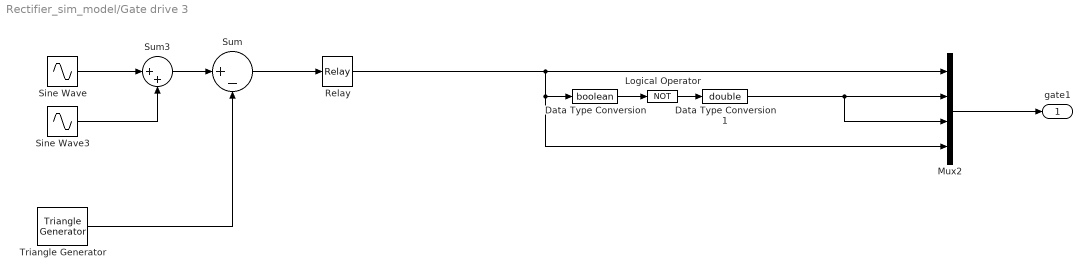
== system Rectifier_sim_model/Gate drive 3 ==
  Data Type Conversion : DataTypeConversion  OutDataTypeStr=boolean
  Data Type Conversion1 : DataTypeConversion  OutDataTypeStr=double
  Logical Operator : Logic  Operator=NOT  AllPortsSameDT=off  OutDataTypeStr=boolean
  Mux2 : Mux
  Relay : Relay
  Sine Wave : Sin  Amplitude=ma1  Frequency=wout  Phase=-2*pi/3+delta  SampleTime=0
  Sine Wave3 : Sin  Amplitude=ma_third  Frequency=f_third*2*pi  Phase=delta_third  SampleTime=0
  Sum : Sum  Inputs=|+-
  Sum3 : Sum  Inputs=|++
  Triangle Generator : powerlib_meascontrol/Pulse & Signal Generators/Triangle Generator  Freq=10000  Phase=0  Ts=Ts
  gate1 : Outport
  wires:
  Sum3/1 -> Sum/1
  Sine Wave3/1 -> Sum3/2
  Sine Wave/1 -> Sum3/1
  Mux2/1 -> gate1/1
  Data Type Conversion1/1 -> Mux2/3, Mux2/2
  Logical Operator/1 -> Data Type Conversion1/1
  Data Type Conversion/1 -> Logical Operator/1
  Sum/1 -> Relay/1
  Triangle Generator/1 -> Sum/2
  Relay/1 -> Mux2/1, Data Type Conversion/1, Mux2/4

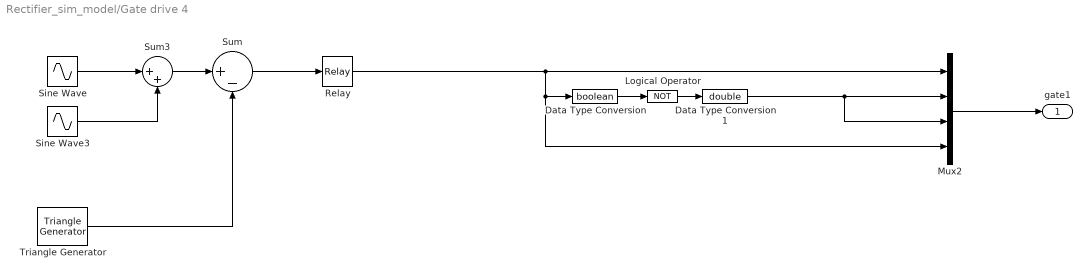
== system Rectifier_sim_model/Gate drive 4 ==
  Data Type Conversion : DataTypeConversion  OutDataTypeStr=boolean
  Data Type Conversion1 : DataTypeConversion  OutDataTypeStr=double
  Logical Operator : Logic  Operator=NOT  AllPortsSameDT=off  OutDataTypeStr=boolean
  Mux2 : Mux
  Relay : Relay
  Sine Wave : Sin  Amplitude=ma1  Frequency=wout  Phase=2*pi/3+delta  SampleTime=0
  Sine Wave3 : Sin  Amplitude=ma_third  Frequency=f_third*2*pi  Phase=delta_third  SampleTime=0
  Sum : Sum  Inputs=|+-
  Sum3 : Sum  Inputs=|++
  Triangle Generator : powerlib_meascontrol/Pulse & Signal Generators/Triangle Generator  Freq=10000  Phase=0  Ts=Ts
  gate1 : Outport
  wires:
  Sum3/1 -> Sum/1
  Sine Wave3/1 -> Sum3/2
  Sine Wave/1 -> Sum3/1
  Mux2/1 -> gate1/1
  Data Type Conversion1/1 -> Mux2/3, Mux2/2
  Logical Operator/1 -> Data Type Conversion1/1
  Data Type Conversion/1 -> Logical Operator/1
  Sum/1 -> Relay/1
  Triangle Generator/1 -> Sum/2
  Relay/1 -> Mux2/1, Data Type Conversion/1, Mux2/4

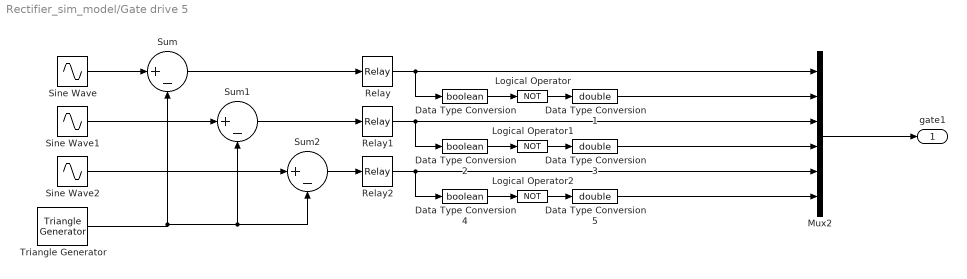
== system Rectifier_sim_model/Gate drive 5 ==
  Data Type Conversion : DataTypeConversion  OutDataTypeStr=boolean
  Data Type Conversion1 : DataTypeConversion  OutDataTypeStr=double
  Data Type Conversion2 : DataTypeConversion  OutDataTypeStr=boolean
  Data Type Conversion3 : DataTypeConversion  OutDataTypeStr=double
  Data Type Conversion4 : DataTypeConversion  OutDataTypeStr=boolean
  Data Type Conversion5 : DataTypeConversion  OutDataTypeStr=double
  Logical Operator : Logic  Operator=NOT  AllPortsSameDT=off  OutDataTypeStr=boolean
  Logical Operator1 : Logic  Operator=NOT  AllPortsSameDT=off  OutDataTypeStr=boolean
  Logical Operator2 : Logic  Operator=NOT  AllPortsSameDT=off  OutDataTypeStr=boolean
  Mux2 : Mux  Inputs=6
  Relay : Relay
  Relay1 : Relay
  Relay2 : Relay
  Sine Wave : Sin  Amplitude=ma1  Frequency=wout  Phase=delta  SampleTime=0
  Sine Wave1 : Sin  Amplitude=ma1  Frequency=wout  Phase=-2*pi/3+delta  SampleTime=0
  Sine Wave2 : Sin  Amplitude=ma1  Frequency=wout  Phase=2*pi/3+delta  SampleTime=0
  Sum : Sum  Inputs=|+-
  Sum1 : Sum  Inputs=|+-
  Sum2 : Sum  Inputs=|+-
  Triangle Generator : powerlib_meascontrol/Pulse & Signal Generators/Triangle Generator  Freq=fsw  Phase=phase(1)  Ts=Ts
  gate1 : Outport
  wires:
  Sine Wave/1 -> Sum/1
  Triangle Generator/1 -> Sum1/2, Sum2/2, Sum/2
  Sine Wave1/1 -> Sum1/1
  Sine Wave2/1 -> Sum2/1
  Sum/1 -> Relay/1
  Sum1/1 -> Relay1/1
  Sum2/1 -> Relay2/1
  Data Type Conversion/1 -> Logical Operator/1
  Relay/1 -> Data Type Conversion/1, Mux2/1
  Logical Operator/1 -> Data Type Conversion1/1
  Data Type Conversion1/1 -> Mux2/2
  Data Type Conversion2/1 -> Logical Operator1/1
  Relay1/1 -> Data Type Conversion2/1, Mux2/3
  Logical Operator1/1 -> Data Type Conversion3/1
  Data Type Conversion3/1 -> Mux2/4
  Data Type Conversion4/1 -> Logical Operator2/1
  Relay2/1 -> Data Type Conversion4/1, Mux2/5
  Logical Operator2/1 -> Data Type Conversion5/1
  Data Type Conversion5/1 -> Mux2/6
  Mux2/1 -> gate1/1

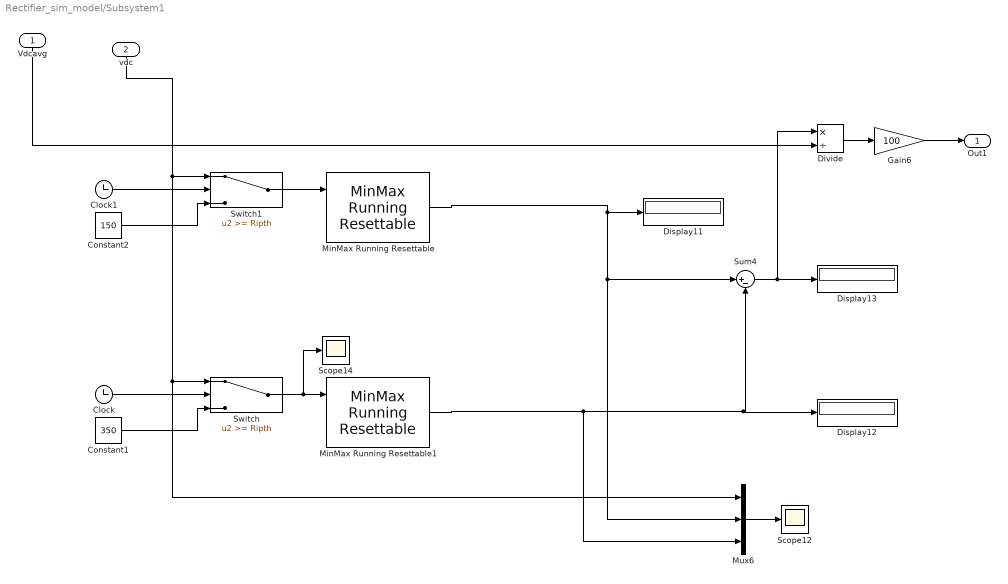
== system Rectifier_sim_model/Subsystem1 ==
  Vdcavg : Inport
  vdc : Inport  Port=2
  Clock : Clock
  Clock1 : Clock
  Constant1 : Constant  Value=350  SampleTime=Ts
  Constant2 : Constant  Value=150  SampleTime=Ts
  Display11 : Display
  Display12 : Display
  Display13 : Display
  Divide : Product  Inputs=*/
  Gain6 : Gain  Gain=100
  MinMax Running Resettable : simulink/Math Operations/MinMax Running Resettable  Function=max  vinit=0.0
  MinMax Running Resettable1 : simulink/Math Operations/MinMax Running Resettable  Function=min  vinit=700
  Mux6 : Mux  Inputs=3
  Scope12 : Scope
  Scope14 : Scope
  Sum4 : Sum  Inputs=|+-
  Switch : Switch  Threshold=Ripth
  Switch1 : Switch  Threshold=Ripth
  Out1 : Outport
  wires:
  MinMax Running Resettable/1 -> Display11/1, Mux6/2, Sum4/1
  Clock/1 -> Switch/2
  Gain6/1 -> Out1/1
  Constant1/1 -> Switch/3
  MinMax Running Resettable1/1 -> Mux6/3, Display12/1, Sum4/2
  Switch/1 -> Scope14/1, MinMax Running Resettable1/1
  Sum4/1 -> Divide/1, Display13/1
  Divide/1 -> Gain6/1
  Mux6/1 -> Scope12/1
  Vdcavg/1 -> Divide/2
  vdc/1 -> Switch1/1, Mux6/1, Switch/1
  Switch1/1 -> MinMax Running Resettable/1
  Clock1/1 -> Switch1/2
  Constant2/1 -> Switch1/3

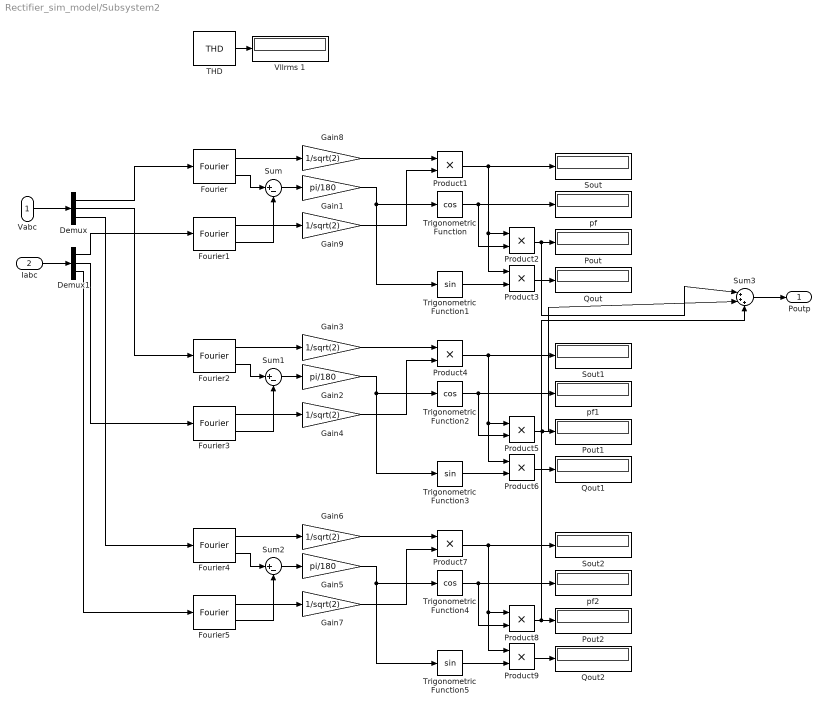
== system Rectifier_sim_model/Subsystem2 ==
  Vabc : Inport
  Iabc : Inport  Port=2
  Demux : Demux  Outputs=3
  Demux1 : Demux  Outputs=3
  Fourier{,1..5} (6 alike) : powerlib_meascontrol/Measurements/Fourier  Freq=fout  n=1  InInit=[0, 0]  Ts=Ts
  Gain1 : Gain  Gain=pi/180
  Gain2 : Gain  Gain=pi/180
  Gain{3..4,6..9} (6 alike) : Gain  Gain=1/sqrt(2)
  Gain5 : Gain  Gain=pi/180
  Pout : Display
  Pout1 : Display
  Pout2 : Display
  Product{1..9} (9 alike) : Product
  Qout : Display
  Qout1 : Display
  Qout2 : Display
  Sout : Display
      settings: Format=short_e
  Sout1 : Display
      settings: Format=short_e
  Sout2 : Display
      settings: Format=short_e
  Sum : Sum  Inputs=|+-
  Sum1 : Sum  Inputs=|+-
  Sum2 : Sum  Inputs=|+-
  Sum3 : Sum  Inputs=|+++
  THD : powerlib_meascontrol/Measurements/THD  Freq=fout  Ts=0
  Trigonometric Function : Trigonometry  Operator=cos
  Trigonometric Function1 : Trigonometry
  Trigonometric Function2 : Trigonometry  Operator=cos
  Trigonometric Function3 : Trigonometry
  Trigonometric Function4 : Trigonometry  Operator=cos
  Trigonometric Function5 : Trigonometry
  Vllrms 1 : Display
  pf : Display
  pf1 : Display
  pf2 : Display
  Poutp : Outport
  wires:
  Gain8/1 -> Product1/1
  Gain9/1 -> Product1/2
  Fourier1/1 -> Gain9/1
  Fourier/1 -> Gain8/1
  Product1/1 -> Product3/1, Product2/1, Sout/1
  Sum/1 -> Gain1/1
  Trigonometric Function/1 -> Product2/2, pf/1
  Gain1/1 -> Trigonometric Function1/1, Trigonometric Function/1
  Product2/1 -> Sum3/1, Pout/1
  THD/1 -> Vllrms 1/1
  Vabc/1 -> Demux/1
  Iabc/1 -> Demux1/1
  Fourier/2 -> Sum/1
  Fourier1/2 -> Sum/2
  Trigonometric Function1/1 -> Product3/2
  Product3/1 -> Qout/1
  Gain3/1 -> Product4/1
  Gain4/1 -> Product4/2
  Fourier3/1 -> Gain4/1
  Fourier2/1 -> Gain3/1
  Product4/1 -> Product6/1, Product5/1, Sout1/1
  Sum1/1 -> Gain2/1
  Trigonometric Function2/1 -> Product5/2, pf1/1
  Gain2/1 -> Trigonometric Function3/1, Trigonometric Function2/1
  Product5/1 -> Sum3/2, Pout1/1
  Fourier2/2 -> Sum1/1
  Fourier3/2 -> Sum1/2
  Trigonometric Function3/1 -> Product6/2
  Product6/1 -> Qout1/1
  Gain6/1 -> Product7/1
  Gain7/1 -> Product7/2
  Fourier5/1 -> Gain7/1
  Fourier4/1 -> Gain6/1
  Product7/1 -> Product9/1, Product8/1, Sout2/1
  Sum2/1 -> Gain5/1
  Trigonometric Function4/1 -> Product8/2, pf2/1
  Gain5/1 -> Trigonometric Function5/1, Trigonometric Function4/1
  Fourier4/2 -> Sum2/1
  Fourier5/2 -> Sum2/2
  Trigonometric Function5/1 -> Product9/2
  Product9/1 -> Qout2/1
  Product8/1 -> Sum3/3, Pout2/1
  Sum3/1 -> Poutp/1
  Demux/1 -> Fourier/1
  Demux/2 -> Fourier2/1
  Demux/3 -> Fourier4/1
  Demux1/1 -> Fourier1/1
  Demux1/2 -> Fourier3/1
  Demux1/3 -> Fourier5/1

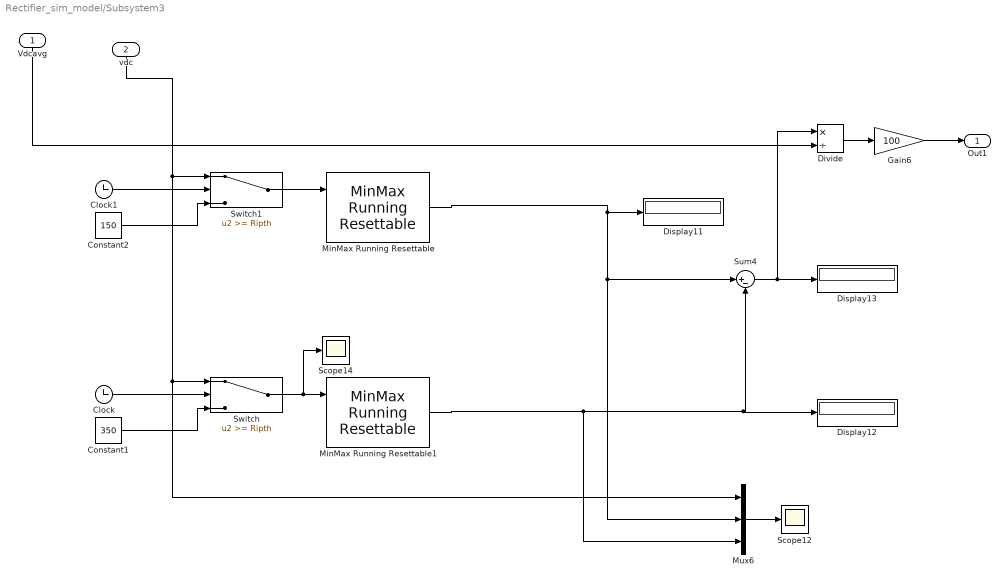
== system Rectifier_sim_model/Subsystem3 ==
  Vdcavg : Inport
  vdc : Inport  Port=2
  Clock : Clock
  Clock1 : Clock
  Constant1 : Constant  Value=350  SampleTime=Ts
  Constant2 : Constant  Value=150  SampleTime=Ts
  Display11 : Display
  Display12 : Display
  Display13 : Display
  Divide : Product  Inputs=*/
  Gain6 : Gain  Gain=100
  MinMax Running Resettable : simulink/Math Operations/MinMax Running Resettable  Function=max  vinit=0.0
  MinMax Running Resettable1 : simulink/Math Operations/MinMax Running Resettable  Function=min  vinit=700
  Mux6 : Mux  Inputs=3
  Scope12 : Scope
  Scope14 : Scope
  Sum4 : Sum  Inputs=|+-
  Switch : Switch  Threshold=Ripth
  Switch1 : Switch  Threshold=Ripth
  Out1 : Outport
  wires:
  MinMax Running Resettable/1 -> Display11/1, Mux6/2, Sum4/1
  Clock/1 -> Switch/2
  Gain6/1 -> Out1/1
  Constant1/1 -> Switch/3
  MinMax Running Resettable1/1 -> Mux6/3, Display12/1, Sum4/2
  Switch/1 -> Scope14/1, MinMax Running Resettable1/1
  Sum4/1 -> Divide/1, Display13/1
  Divide/1 -> Gain6/1
  Mux6/1 -> Scope12/1
  Vdcavg/1 -> Divide/2
  vdc/1 -> Switch1/1, Mux6/1, Switch/1
  Switch1/1 -> MinMax Running Resettable/1
  Clock1/1 -> Switch1/2
  Constant2/1 -> Switch1/3

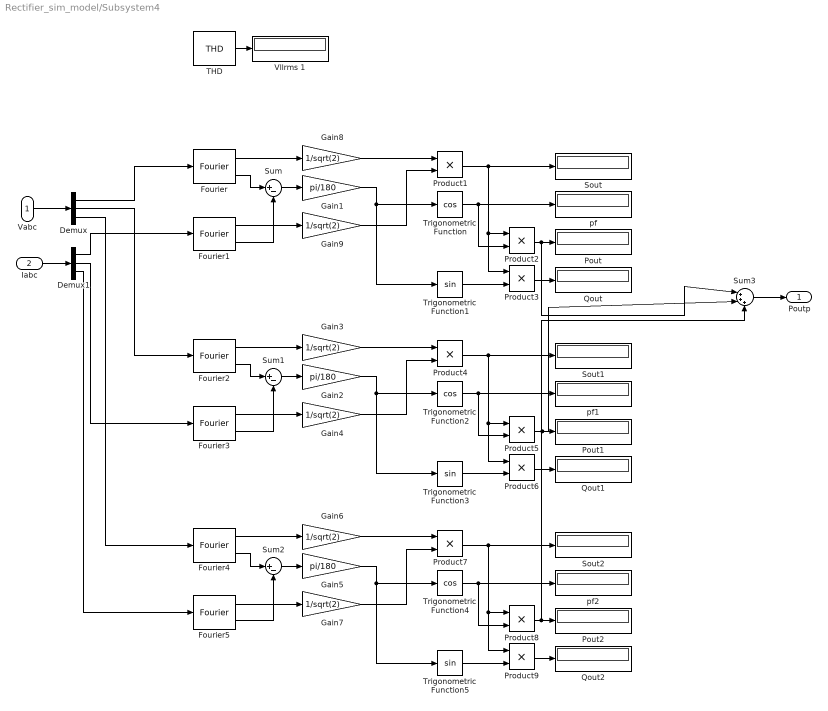
== system Rectifier_sim_model/Subsystem4 ==
  Vabc : Inport
  Iabc : Inport  Port=2
  Demux : Demux  Outputs=3
  Demux1 : Demux  Outputs=3
  Fourier{,1..5} (6 alike) : powerlib_meascontrol/Measurements/Fourier  Freq=fout  n=1  InInit=[0, 0]  Ts=Ts
  Gain1 : Gain  Gain=pi/180
  Gain2 : Gain  Gain=pi/180
  Gain{3..4,6..9} (6 alike) : Gain  Gain=1/sqrt(2)
  Gain5 : Gain  Gain=pi/180
  Pout : Display
  Pout1 : Display
  Pout2 : Display
  Product{1..9} (9 alike) : Product
  Qout : Display
  Qout1 : Display
  Qout2 : Display
  Sout : Display
      settings: Format=short_e
  Sout1 : Display
      settings: Format=short_e
  Sout2 : Display
      settings: Format=short_e
  Sum : Sum  Inputs=|+-
  Sum1 : Sum  Inputs=|+-
  Sum2 : Sum  Inputs=|+-
  Sum3 : Sum  Inputs=|+++
  THD : powerlib_meascontrol/Measurements/THD  Freq=fout  Ts=0
  Trigonometric Function : Trigonometry  Operator=cos
  Trigonometric Function1 : Trigonometry
  Trigonometric Function2 : Trigonometry  Operator=cos
  Trigonometric Function3 : Trigonometry
  Trigonometric Function4 : Trigonometry  Operator=cos
  Trigonometric Function5 : Trigonometry
  Vllrms 1 : Display
  pf : Display
  pf1 : Display
  pf2 : Display
  Poutp : Outport
  wires:
  Gain8/1 -> Product1/1
  Gain9/1 -> Product1/2
  Fourier1/1 -> Gain9/1
  Fourier/1 -> Gain8/1
  Product1/1 -> Product3/1, Product2/1, Sout/1
  Sum/1 -> Gain1/1
  Trigonometric Function/1 -> Product2/2, pf/1
  Gain1/1 -> Trigonometric Function1/1, Trigonometric Function/1
  Product2/1 -> Sum3/1, Pout/1
  THD/1 -> Vllrms 1/1
  Vabc/1 -> Demux/1
  Iabc/1 -> Demux1/1
  Fourier/2 -> Sum/1
  Fourier1/2 -> Sum/2
  Trigonometric Function1/1 -> Product3/2
  Product3/1 -> Qout/1
  Gain3/1 -> Product4/1
  Gain4/1 -> Product4/2
  Fourier3/1 -> Gain4/1
  Fourier2/1 -> Gain3/1
  Product4/1 -> Product6/1, Product5/1, Sout1/1
  Sum1/1 -> Gain2/1
  Trigonometric Function2/1 -> Product5/2, pf1/1
  Gain2/1 -> Trigonometric Function3/1, Trigonometric Function2/1
  Product5/1 -> Sum3/2, Pout1/1
  Fourier2/2 -> Sum1/1
  Fourier3/2 -> Sum1/2
  Trigonometric Function3/1 -> Product6/2
  Product6/1 -> Qout1/1
  Gain6/1 -> Product7/1
  Gain7/1 -> Product7/2
  Fourier5/1 -> Gain7/1
  Fourier4/1 -> Gain6/1
  Product7/1 -> Product9/1, Product8/1, Sout2/1
  Sum2/1 -> Gain5/1
  Trigonometric Function4/1 -> Product8/2, pf2/1
  Gain5/1 -> Trigonometric Function5/1, Trigonometric Function4/1
  Fourier4/2 -> Sum2/1
  Fourier5/2 -> Sum2/2
  Trigonometric Function5/1 -> Product9/2
  Product9/1 -> Qout2/1
  Product8/1 -> Sum3/3, Pout2/1
  Sum3/1 -> Poutp/1
  Demux/1 -> Fourier/1
  Demux/2 -> Fourier2/1
  Demux/3 -> Fourier4/1
  Demux1/1 -> Fourier1/1
  Demux1/2 -> Fourier3/1
  Demux1/3 -> Fourier5/1

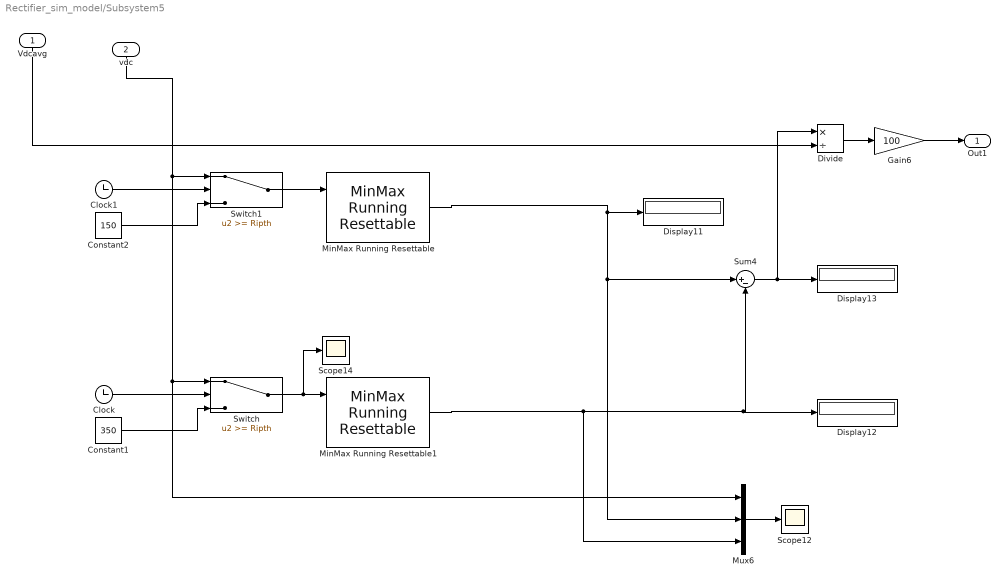
== system Rectifier_sim_model/Subsystem5 ==
  Vdcavg : Inport
  vdc : Inport  Port=2
  Clock : Clock
  Clock1 : Clock
  Constant1 : Constant  Value=350  SampleTime=Ts
  Constant2 : Constant  Value=150  SampleTime=Ts
  Display11 : Display
  Display12 : Display
  Display13 : Display
  Divide : Product  Inputs=*/
  Gain6 : Gain  Gain=100
  MinMax Running Resettable : simulink/Math Operations/MinMax Running Resettable  Function=max  vinit=0.0
  MinMax Running Resettable1 : simulink/Math Operations/MinMax Running Resettable  Function=min  vinit=700
  Mux6 : Mux  Inputs=3
  Scope12 : Scope
  Scope14 : Scope
  Sum4 : Sum  Inputs=|+-
  Switch : Switch  Threshold=Ripth
  Switch1 : Switch  Threshold=Ripth
  Out1 : Outport
  wires:
  MinMax Running Resettable/1 -> Display11/1, Mux6/2, Sum4/1
  Clock/1 -> Switch/2
  Gain6/1 -> Out1/1
  Constant1/1 -> Switch/3
  MinMax Running Resettable1/1 -> Mux6/3, Display12/1, Sum4/2
  Switch/1 -> Scope14/1, MinMax Running Resettable1/1
  Sum4/1 -> Divide/1, Display13/1
  Divide/1 -> Gain6/1
  Mux6/1 -> Scope12/1
  Vdcavg/1 -> Divide/2
  vdc/1 -> Switch1/1, Mux6/1, Switch/1
  Switch1/1 -> MinMax Running Resettable/1
  Clock1/1 -> Switch1/2
  Constant2/1 -> Switch1/3

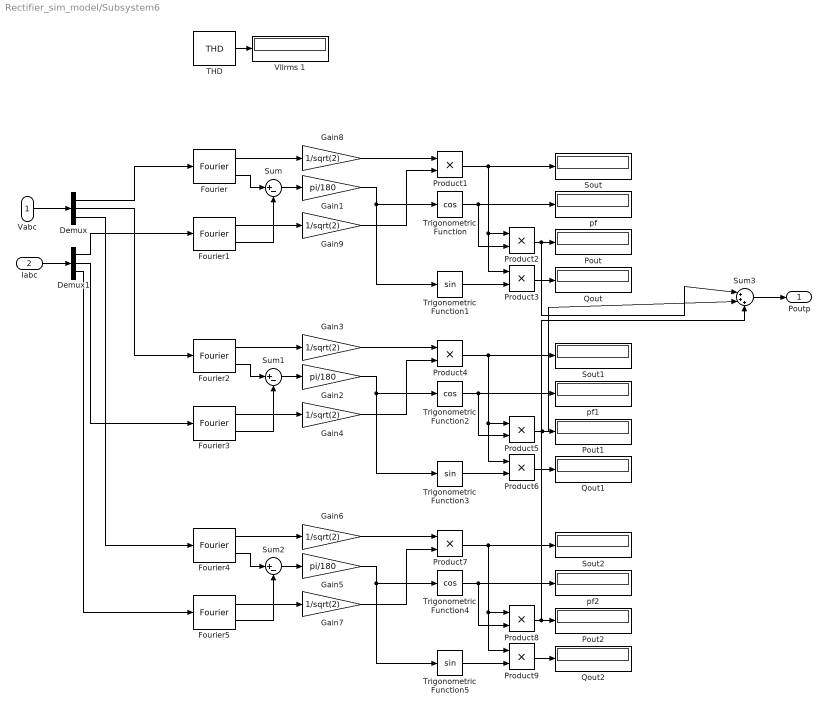
== system Rectifier_sim_model/Subsystem6 ==
  Vabc : Inport
  Iabc : Inport  Port=2
  Demux : Demux  Outputs=3
  Demux1 : Demux  Outputs=3
  Fourier{,1..5} (6 alike) : powerlib_meascontrol/Measurements/Fourier  Freq=fout  n=1  InInit=[0, 0]  Ts=Ts
  Gain1 : Gain  Gain=pi/180
  Gain2 : Gain  Gain=pi/180
  Gain{3..4,6..9} (6 alike) : Gain  Gain=1/sqrt(2)
  Gain5 : Gain  Gain=pi/180
  Pout : Display
  Pout1 : Display
  Pout2 : Display
  Product{1..9} (9 alike) : Product
  Qout : Display
  Qout1 : Display
  Qout2 : Display
  Sout : Display
      settings: Format=short_e
  Sout1 : Display
      settings: Format=short_e
  Sout2 : Display
      settings: Format=short_e
  Sum : Sum  Inputs=|+-
  Sum1 : Sum  Inputs=|+-
  Sum2 : Sum  Inputs=|+-
  Sum3 : Sum  Inputs=|+++
  THD : powerlib_meascontrol/Measurements/THD  Freq=fout  Ts=0
  Trigonometric Function : Trigonometry  Operator=cos
  Trigonometric Function1 : Trigonometry
  Trigonometric Function2 : Trigonometry  Operator=cos
  Trigonometric Function3 : Trigonometry
  Trigonometric Function4 : Trigonometry  Operator=cos
  Trigonometric Function5 : Trigonometry
  Vllrms 1 : Display
  pf : Display
  pf1 : Display
  pf2 : Display
  Poutp : Outport
  wires:
  Gain8/1 -> Product1/1
  Gain9/1 -> Product1/2
  Fourier1/1 -> Gain9/1
  Fourier/1 -> Gain8/1
  Product1/1 -> Product3/1, Product2/1, Sout/1
  Sum/1 -> Gain1/1
  Trigonometric Function/1 -> Product2/2, pf/1
  Gain1/1 -> Trigonometric Function1/1, Trigonometric Function/1
  Product2/1 -> Sum3/1, Pout/1
  THD/1 -> Vllrms 1/1
  Vabc/1 -> Demux/1
  Iabc/1 -> Demux1/1
  Fourier/2 -> Sum/1
  Fourier1/2 -> Sum/2
  Trigonometric Function1/1 -> Product3/2
  Product3/1 -> Qout/1
  Gain3/1 -> Product4/1
  Gain4/1 -> Product4/2
  Fourier3/1 -> Gain4/1
  Fourier2/1 -> Gain3/1
  Product4/1 -> Product6/1, Product5/1, Sout1/1
  Sum1/1 -> Gain2/1
  Trigonometric Function2/1 -> Product5/2, pf1/1
  Gain2/1 -> Trigonometric Function3/1, Trigonometric Function2/1
  Product5/1 -> Sum3/2, Pout1/1
  Fourier2/2 -> Sum1/1
  Fourier3/2 -> Sum1/2
  Trigonometric Function3/1 -> Product6/2
  Product6/1 -> Qout1/1
  Gain6/1 -> Product7/1
  Gain7/1 -> Product7/2
  Fourier5/1 -> Gain7/1
  Fourier4/1 -> Gain6/1
  Product7/1 -> Product9/1, Product8/1, Sout2/1
  Sum2/1 -> Gain5/1
  Trigonometric Function4/1 -> Product8/2, pf2/1
  Gain5/1 -> Trigonometric Function5/1, Trigonometric Function4/1
  Fourier4/2 -> Sum2/1
  Fourier5/2 -> Sum2/2
  Trigonometric Function5/1 -> Product9/2
  Product9/1 -> Qout2/1
  Product8/1 -> Sum3/3, Pout2/1
  Sum3/1 -> Poutp/1
  Demux/1 -> Fourier/1
  Demux/2 -> Fourier2/1
  Demux/3 -> Fourier4/1
  Demux1/1 -> Fourier1/1
  Demux1/2 -> Fourier3/1
  Demux1/3 -> Fourier5/1
